simulink model "am"  (R2023b)
settings: Solver=VariableStepAuto  StartTime=0.0  StopTime=10.0  RelTol=1e-3
settings Model: Creator=ASUS  LastModifiedBy=ASUS

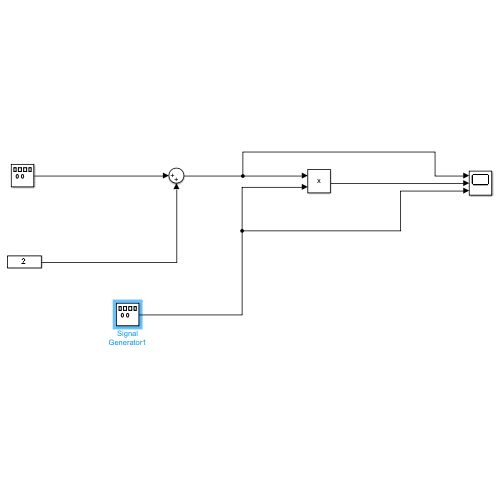
[thumbnail: Simulink's stored preview of the top-level diagram]
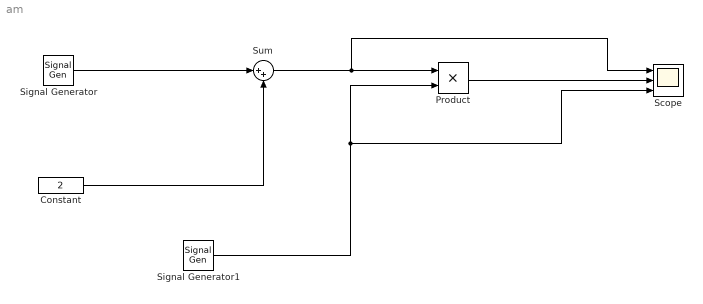
== system am ==
  Constant : Constant  Value=2  SampleTime=0.01
  Product : Product
  Scope : Scope  NumInputPorts=3
  Signal Generator : SignalGenerator  Amplitude=3  Frequency=3  Units=rad/sec
  Signal Generator1 : SignalGenerator  Amplitude=2  Frequency=100  Units=rad/sec
  Sum : Sum  Inputs=|++
  wires:
  Signal Generator/1 -> Sum/1
  Constant/1 -> Sum/2
  Signal Generator1/1 -> Scope/3, Product/2
  Sum/1 -> Scope/1, Product/1
  Product/1 -> Scope/2
